simulink model "case123_simulink"  (R2015b)
settings: Solver=FixedStepAuto  StartTime=12  StopTime=123.2400  FixedStep=.02  RelTol=1e-3
values from neighbouring files (symbols this model uses):
  c2 = 2    [Project1_Guilherme_Mollica.m]    (also in myfun.m; myfunnon.m; num3.m = damp; num3_30deg.m = damp)
settings Model: Creator=guilh_000  LastModifiedBy=guilh_000

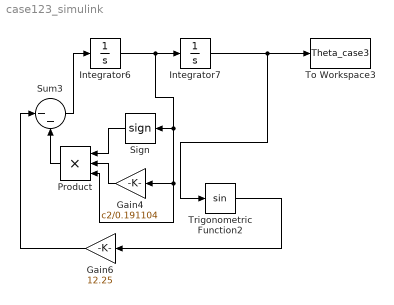
== system case123_simulink ==
  Gain4 : Gain  Gain=c2/0.191104
  Gain6 : Gain  Gain=12.25
  Integrator6 : Integrator
  Integrator7 : Integrator  InitialCondition=-pi/4
  Product : Product  Inputs=3
  Sign : Signum
  Sum3 : Sum  Inputs=|--
  To Workspace3 : ToWorkspace  VariableName=Theta_case3  SampleTime=-1
  Trigonometric Function2 : Trigonometry
  wires:
  Sum3/1 -> Integrator6/1
  Gain6/1 -> Sum3/1
  Integrator7/1 -> Trigonometric Function2/1, To Workspace3/1
  Trigonometric Function2/1 -> Gain6/1
  Product/1 -> Sum3/2
  Sign/1 -> Product/1
  Gain4/1 -> Product/2
  Integrator6/1 -> Product/3, Gain4/1, Sign/1, Integrator7/1
